simulink model "simulink1"  (Simulink 7.9)
settings: Solver=ode45  StartTime=0.0  StopTime=10.0  RelTol=1e-3
libraries: simulink x2
settings Model: Creator=SzLidia  LastModifiedBy=SzLidia

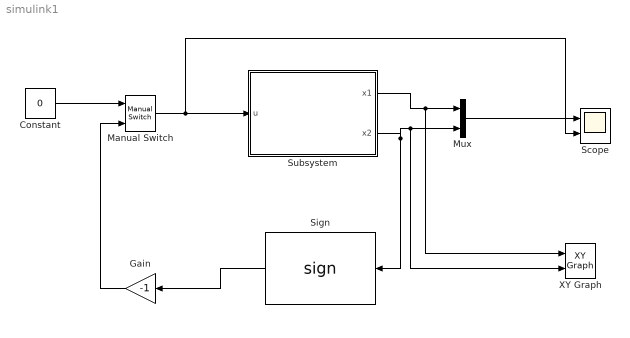
== system simulink1 ==
  Constant : Constant  Value=0  SampleTime=-1
  Gain : Gain  Gain=-1
  Manual Switch : simulink/Signal Routing/Manual Switch  sw=0  action=0  varsize=off
  Mux : Mux  Inputs=2
  Scope : Scope  NumInputPorts=2
      settings: YMin=-5~-5  YMax=5~5
  Sign : Signum
  Subsystem : Subsystem  mask{w=5, x0=[2, 3]}
  XY Graph : simulink/Sinks/XY Graph  xmin=-1  xmax=1  ymin=-1  ymax=1  st=0.001
  wires:
  Constant/1 -> Manual Switch/1
  Manual Switch/1 -> Subsystem/1(u), Scope/2
  Subsystem/1(x1) -> Mux/1, XY Graph/1
  Mux/1 -> Scope/1
  Gain/1 -> Manual Switch/2
  Sign/1 -> Gain/1
  Subsystem/2(x2) -> Sign/1, Mux/2, XY Graph/2

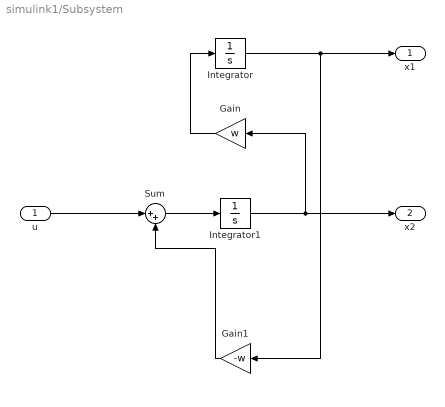
== system simulink1/Subsystem ==
  u : Inport
  Gain : Gain  Gain=w
  Gain1 : Gain  Gain=-w
  Integrator : Integrator  InitialCondition=x0(1)
  Integrator1 : Integrator  InitialCondition=x0(2)
  Sum : Sum  Inputs=|++
  x1 : Outport
  x2 : Outport  Port=2
  wires:
  Integrator/1 -> x1/1, Gain1/1
  Integrator1/1 -> x2/1, Gain/1
  u/1 -> Sum/1
  Sum/1 -> Integrator1/1
  Gain1/1 -> Sum/2
  Gain/1 -> Integrator/1
